simulink model "4_4PVstring"  (R2023b)
settings: Solver=ode3  StartTime=0.0  StopTime=0.25  FixedStep=1e-5  RelTol=1e-3
libraries: spsDiodeLib x16, spsPVArrayLib x16, spsControlledVoltageSourceLib x1, spsCurrentMeasurementLib x1, simulink x1, spsVoltageMeasurementLib x1, sps_lib x1
settings Model: Creator=ameen  LastModifiedBy=ameen

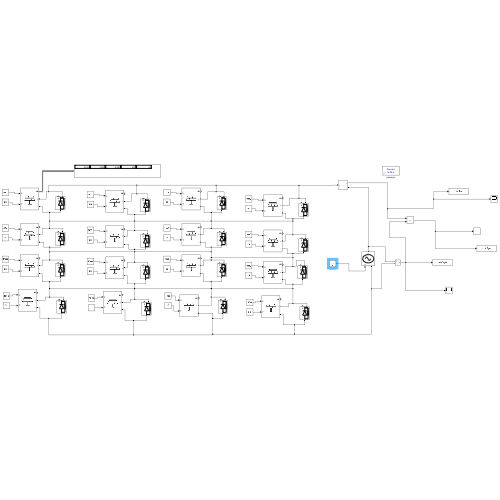
[thumbnail: Simulink's stored preview of the top-level diagram]
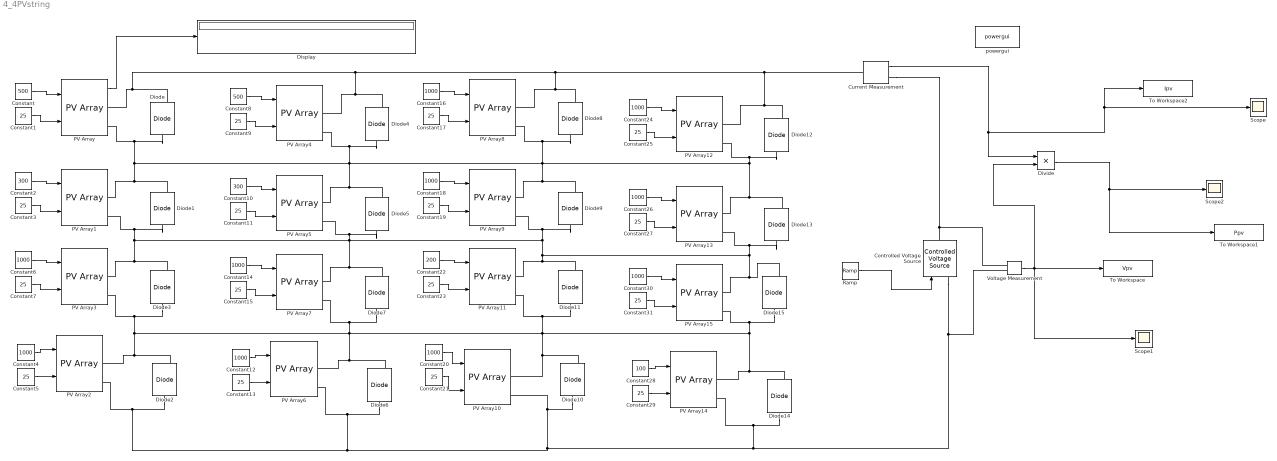
== system 4_4PVstring ==
  Constant : Constant  Value=500
  Constant{1,3,5,7,9,11,13,15,17,19,21,23,25,27,29,31} (16 alike) : Constant  Value=25
  Constant10 : Constant  Value=300
  Constant{4,6,12,14,16,18,20,24,26,30} (10 alike) : Constant  Value=1000
  Constant2 : Constant  Value=300
  Constant22 : Constant  Value=200
  Constant28 : Constant  Value=100
  Constant8 : Constant  Value=500
  Controlled Voltage Source : spsControlledVoltageSourceLib/Controlled Voltage Source  Initialize=on  Source_Type=AC  Amplitude=0  Phase=0  Frequency=0  Measurements=None
  Current Measurement : spsCurrentMeasurementLib/Current Measurement  PhasorSimulation=off  OutputType=Complex  PSBequivalent=0
  Diode{,1..15} (16 alike) : spsDiodeLib/Diode  Ron=0.001  Lon=0  Vf=0.8  IC=0  UseSnubber=0  Rs=500  Cs=250e-9  Measurements=on
  Display : Display
  Divide : Product  RndMeth=Zero  SaturateOnIntegerOverflow=on
  PV Array{,1..15} (16 alike) : spsPVArrayLib/PV Array  Npar=1  Nser=1  PlotType=array @ 25 deg.C & specified irradiances  S_vec="[ 1000  500  100 ]"  Temp_C_vec="[ 45 25  ]"  ModuleName=User-defined  PlotWhenSelected=off  Pm=213.15  Ncell=60  Voc=36.3  Isc=7.84  Vm=29  Im=7.35  beta_Voc_pc=-0.36099  alpha_Isc_pc=0.102  beta_Voc=-0.13104  alpha_Isc=0.0079968  IL=7.8654  I0=2.9273e-10  nI=0.98119  Rsh=313.0553  Rs=0.39381  RobustModel=off  RobustCellTemperature=313.3991  BAL=off  Tc=1e-6  Tfilter=1e-5
  Ramp : simulink/Sources/Ramp  slope=36.3*4*4  start=0  InitialOutput=0
  Scope : Scope
  Scope1 : Scope
  Scope2 : Scope
  To Workspace : ToWorkspace  VariableName=Vpv  SaveFormat=Structure With Time  SampleTime=-1
  To Workspace1 : ToWorkspace  VariableName=Ppv  SaveFormat=Structure With Time  SampleTime=-1
  To Workspace2 : ToWorkspace  VariableName=Ipv  SaveFormat=Structure With Time  SampleTime=-1
  Voltage Measurement : spsVoltageMeasurementLib/Voltage Measurement  PhasorSimulation=off  OutputType=Complex  PSBequivalent=0
  powergui : sps_lib/powergui  Priority=1  SimulationMode=Discrete  SampleTime=1e-5  frequency=60  Iterations=50  frequencyindice=0  Pbase=100e6  ErrMax=1e-4  UnitsV=kV  UnitsW=MW  buscounter=0  FunctionMessages=off  echomessages=off  EnableUseOfTLC=off  CurrentSourceSwitches=off  DisableSnubberDevices=off  DisableRonSwitches=off  DisableVfSwitches=off  DisplayEquations=off  AutomaticDiscreteSolvers=off  SolverType=Tustin  Interpol=off  ExternalGateDelay=off  methode=off  Ts=100  x0status=blocks  SPID=on  SwTol=0  HookPort=off  NonlinearTolerance=1e-4  nMaxIteration=100  ContinueOnMaxIteration=off  RestoreLinks=warning  ResistiveCurrentMeasurement=off  Frange=[0:2:500]  Ylog=off  Xlog=on  ShowGrid=off  save=off  variable=ZData  structure=0  ZoomFFT=off  StartTime=0.0  cycles=1  DisplayStyle=1  fundamental=60  FreqAxis=off  MaxFrequency=1000  frequencyindicesteady=1  RmsSteady=1  display=off
  wires:
  Constant/1 -> PV Array/1
  Constant1/1 -> PV Array/2
  Constant3/1 -> PV Array1/2
  Constant2/1 -> PV Array1/1
  Constant5/1 -> PV Array2/2
  Constant4/1 -> PV Array2/1
  Constant7/1 -> PV Array3/2
  Constant6/1 -> PV Array3/1
  Constant15/1 -> PV Array7/2
  Constant12/1 -> PV Array6/1
  Constant13/1 -> PV Array6/2
  Constant14/1 -> PV Array7/1
  Constant11/1 -> PV Array5/2
  Constant9/1 -> PV Array4/2
  Constant8/1 -> PV Array4/1
  Constant10/1 -> PV Array5/1
  Constant23/1 -> PV Array11/2
  Constant20/1 -> PV Array10/1
  Constant21/1 -> PV Array10/2
  Constant22/1 -> PV Array11/1
  Constant19/1 -> PV Array9/2
  Constant17/1 -> PV Array8/2
  Constant16/1 -> PV Array8/1
  Constant18/1 -> PV Array9/1
  Constant31/1 -> PV Array15/2
  Constant28/1 -> PV Array14/1
  Constant29/1 -> PV Array14/2
  Constant30/1 -> PV Array15/1
  Constant27/1 -> PV Array13/2
  Constant25/1 -> PV Array12/2
  Constant24/1 -> PV Array12/1
  Constant26/1 -> PV Array13/1
  Ramp/1 -> Controlled Voltage Source/1
  Current Measurement/1 -> Scope/1, To Workspace2/1, Divide/1
  Voltage Measurement/1 -> Divide/2, Scope1/1, To Workspace/1
  Divide/1 -> To Workspace1/1, Scope2/1
  PV Array/1 -> Display/1
  connections:
  Diode3/LConn1 -- PV Array3/RConn2 -- PV Array2/RConn1 -- Diode2/RConn1 -- PV Array7/RConn2 -- Diode7/LConn1 -- PV Array10/RConn1 -- Diode10/RConn1 -- PV Array14/RConn1 -- Diode14/RConn1 -- PV Array15/RConn2 -- Diode15/LConn1 -- PV Array11/RConn2 -- Diode11/LConn1 -- PV Array6/RConn1 -- Diode6/RConn1
  Diode1/LConn1 -- PV Array1/RConn2 -- PV Array3/RConn1 -- Diode3/RConn1 -- PV Array7/RConn1 -- Diode7/RConn1 -- PV Array5/RConn2 -- Diode5/LConn1 -- PV Array15/RConn1 -- Diode15/RConn1 -- PV Array13/RConn2 -- Diode13/LConn1 -- PV Array11/RConn1 -- Diode11/RConn1 -- PV Array9/RConn2 -- Diode9/LConn1
  Diode/LConn1 -- PV Array/RConn2 -- PV Array9/RConn1 -- Diode9/RConn1 -- PV Array13/RConn1 -- Diode13/RConn1 -- PV Array12/RConn2 -- Diode12/LConn1 -- PV Array8/RConn2 -- Diode8/LConn1 -- PV Array5/RConn1 -- Diode5/RConn1 -- PV Array4/RConn2 -- Diode4/LConn1 -- PV Array1/RConn1 -- Diode1/RConn1
  Diode2/LConn1 -- Voltage Measurement/LConn2 -- Controlled Voltage Source/LConn1 -- PV Array14/RConn2 -- Diode14/LConn1 -- PV Array10/RConn2 -- Diode10/LConn1 -- PV Array6/RConn2 -- Diode6/LConn1 -- PV Array2/RConn2
  Diode/RConn1 -- PV Array12/RConn1 -- Diode12/RConn1 -- Current Measurement/LConn1 -- PV Array8/RConn1 -- Diode8/RConn1 -- PV Array4/RConn1 -- Diode4/RConn1 -- PV Array/RConn1
  Current Measurement/RConn1 -- Voltage Measurement/LConn1 -- Controlled Voltage Source/RConn1
